simulink model "umbral_adaptativo_prueba"  (R2018a)
settings: Solver=VariableStepAuto  StartTime=0.0  StopTime=10.0  RelTol=1e-3
settings Model: Creator=carma  LastModifiedBy=carma

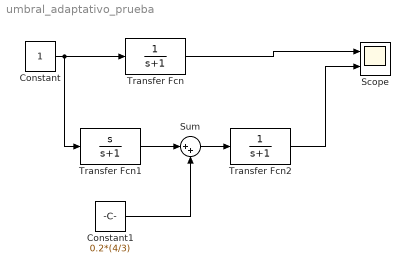
== system umbral_adaptativo_prueba ==
  Constant : Constant
  Constant1 : Constant  Value=0.2*(4/3)
  Scope : Scope  NumInputPorts=2
  Sum : Sum  Inputs=|++
  Transfer Fcn : TransferFcn  Denominator=[1 1]
  Transfer Fcn1 : TransferFcn  Numerator=[1 0]  Denominator=[1 1]
  Transfer Fcn2 : TransferFcn  Denominator=[1 1]
  wires:
  Constant/1 -> Transfer Fcn1/1, Transfer Fcn/1
  Transfer Fcn/1 -> Scope/1
  Constant1/1 -> Sum/2
  Transfer Fcn1/1 -> Sum/1
  Sum/1 -> Transfer Fcn2/1
  Transfer Fcn2/1 -> Scope/2
